simulink model "prog_control2610"  (R2024a)
settings: Solver=VariableStepAuto  StartTime=0.0  StopTime=14  RelTol=1e-3
settings Model: Creator=pupkinzalupkin  LastModifiedBy=pupkinzalupkin

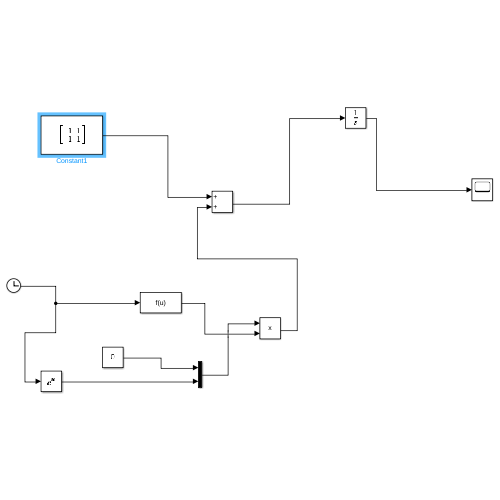
[thumbnail: Simulink's stored preview of the top-level diagram]
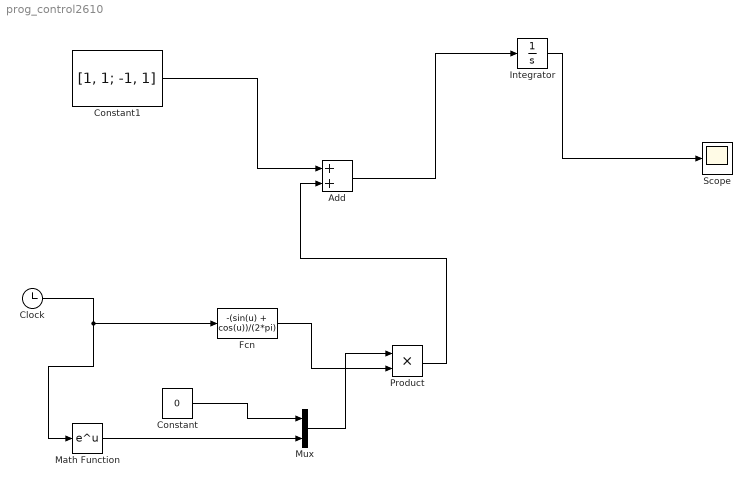
== system prog_control2610 ==
  Add : Sum
  Clock : Clock
  Constant : Constant  Value=0
  Constant1 : Constant  Value=[1, 1; -1, 1]
  Fcn : Fcn  Expr=-(sin(u) + cos(u))/(2*pi)
  Integrator : Integrator  InitialCondition=[-1; -1]
  Math Function : Math
  Mux : Mux  Inputs=2
  Product : Product
  Scope : Scope
  wires:
  Integrator/1 -> Scope/1
  Clock/1 -> Fcn/1, Math Function/1
  Mux/1 -> Product/1
  Fcn/1 -> Product/2
  Math Function/1 -> Mux/2
  Constant/1 -> Mux/1
  Product/1 -> Add/2
  Constant1/1 -> Add/1
  Add/1 -> Integrator/1
